simulink library "LiBatteryBlocks"  (Simulink 7.6)
settings: Solver=ode45  StartTime=0.0  StopTime=10.0  RelTol=1e-3
values from neighbouring files (symbols this model uses):
  BatteryParams = struct()    [ssc_lithium_battery_80Cells_ini.m]
  numCells = 80    [ssc_lithium_battery_80Cells_ini.m]
libraries: fl_lib x19, LiBatteryBlocks x8, LiBatteryElements_lib x4, nesl_utility x3
settings Model: Creator=jgazzarr  LastModifiedBy=rjackey

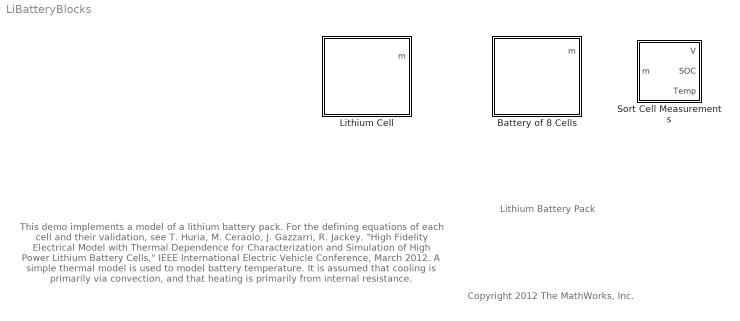
== system LiBatteryBlocks ==
  note: Lithium Battery Pack
  note: This demo implements a model of a lithium battery pack. For the defining equations of each cell and their validation, see T. Huria, M. Ceraolo,
      | J. Gazzarri, R. Jackey. "High Fidelity Electrical Model with Thermal Dependence for Characterization and Simulation of High Power Lithium
      | Battery Cells," IEEE International Electric Vehicle Conference, March 2012. A simple thermal model is used to model battery temperature. It is
      | assumed that cooling is primarily via convection, and that heating is primarily from internal resistance.
  note: Copyright 2012 The MathWorks, Inc.
  Battery of 8 Cells : Subsystem  mask(Battery 8 Series Cells){ThisStackParams=BatteryParams(1:8)}
      mask prompts: ThisStackParams "Parameter Structure (this stack of cells)"
      settings: AttributesFormatString=%<ThisStackParams>
  Lithium Cell : Subsystem  mask(Battery Cell){Battery=BatteryParams(1)}
      mask prompts: Battery "Battery Parameter Structure"
      settings: AttributesFormatString=%<Battery>
      mask Display:
      | image(imread('battery.jpg'))
      | color('red')
      | port_label('LConn',2,'-')
      | port_label('LConn',1,'+')
      | port_label('RConn',1,'H')
      | port_label('output',1,'m')
  Sort Cell Measurements : Subsystem

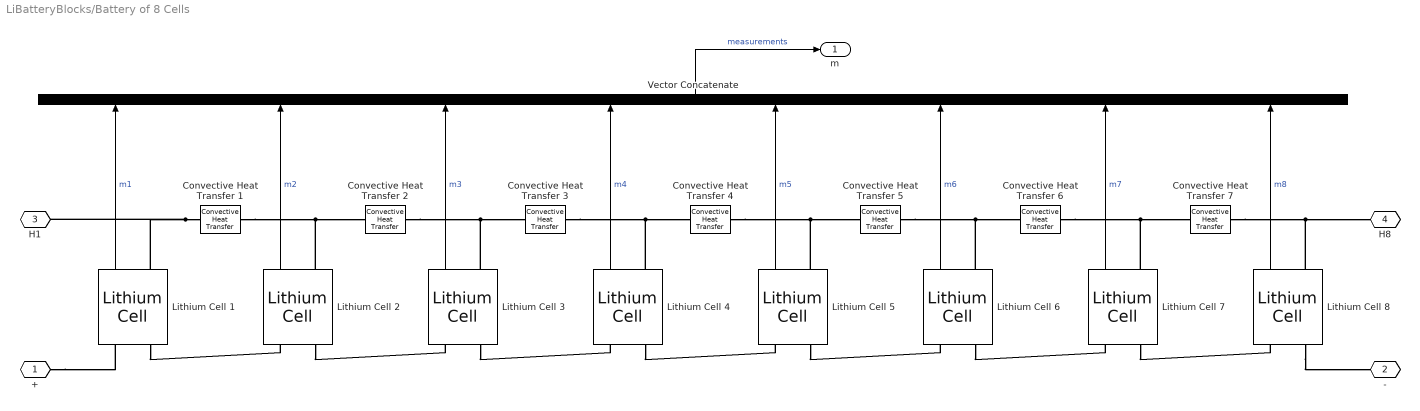
== system LiBatteryBlocks/Battery of 8 Cells ==
  Convective Heat Transfer {1..7} (7 alike) : fl_lib/Thermal/Thermal Elements/Convective Heat Transfer  DialogController=NetworkEngine.DynNeDlgSource  SystemSampleTime=-1  area=cell_area m^2  heat_tr_coeff=h_conv W/(m^2 * K)  Q_Log=off  T_Log=off  LocalVarNames=|heat_flow|temperature_diff  LocalVarDescs=|Heat flow (J/s)|Temperature difference (K)  LocalVarLogging=[0 0]
  Lithium Cell 1 : LiBatteryBlocks/Lithium Cell  SystemSampleTime=-1  Battery=ThisStackParams(1)
      settings: AttributesFormatString=%<Battery>
  Lithium Cell 2 : LiBatteryBlocks/Lithium Cell  SystemSampleTime=-1  Battery=ThisStackParams(2)
      settings: AttributesFormatString=%<Battery>
  Lithium Cell 3 : LiBatteryBlocks/Lithium Cell  SystemSampleTime=-1  Battery=BatteryParams(3)
      settings: AttributesFormatString=%<Battery>
  Lithium Cell 4 : LiBatteryBlocks/Lithium Cell  SystemSampleTime=-1  Battery=ThisStackParams(4)
      settings: AttributesFormatString=%<Battery>
  Lithium Cell 5 : LiBatteryBlocks/Lithium Cell  SystemSampleTime=-1  Battery=ThisStackParams(5)
      settings: AttributesFormatString=%<Battery>
  Lithium Cell 6 : LiBatteryBlocks/Lithium Cell  SystemSampleTime=-1  Battery=ThisStackParams(6)
      settings: AttributesFormatString=%<Battery>
  Lithium Cell 7 : LiBatteryBlocks/Lithium Cell  SystemSampleTime=-1  Battery=ThisStackParams(7)
      settings: AttributesFormatString=%<Battery>
  Lithium Cell 8 : LiBatteryBlocks/Lithium Cell  SystemSampleTime=-1  Battery=ThisStackParams(8)
      settings: AttributesFormatString=%<Battery>
  Vector Concatenate : Concatenate  NumInputs=8  Mode=Vector
  + : PMIOPort  Port=1  Side=Left
  - : PMIOPort  Port=2  Side=Left
  H1 : PMIOPort  Port=3  Side=Right
  H8 : PMIOPort  Port=4  Side=Right
  m : Outport
  wires:
  Lithium Cell 1/1 -> Vector Concatenate/1  "m1"
  Lithium Cell 2/1 -> Vector Concatenate/2  "m2"
  Lithium Cell 3/1 -> Vector Concatenate/3  "m3"
  Lithium Cell 4/1 -> Vector Concatenate/4  "m4"
  Lithium Cell 5/1 -> Vector Concatenate/5  "m5"
  Lithium Cell 6/1 -> Vector Concatenate/6  "m6"
  Lithium Cell 7/1 -> Vector Concatenate/7  "m7"
  Lithium Cell 8/1 -> Vector Concatenate/8  "m8"
  Vector Concatenate/1 -> m/1  "measurements"
  connections:
  Lithium Cell 8/RConn1 -- H8/RConn1 -- Convective Heat Transfer 7/RConn1
  Convective Heat Transfer 1/LConn1 -- H1/RConn1 -- Lithium Cell 1/RConn1
  Lithium Cell 7/LConn2 -- Lithium Cell 8/LConn1
  Lithium Cell 6/LConn2 -- Lithium Cell 7/LConn1
  Lithium Cell 5/LConn2 -- Lithium Cell 6/LConn1
  Lithium Cell 4/LConn2 -- Lithium Cell 5/LConn1
  Lithium Cell 3/LConn2 -- Lithium Cell 4/LConn1
  Lithium Cell 2/LConn2 -- Lithium Cell 3/LConn1
  Lithium Cell 1/LConn2 -- Lithium Cell 2/LConn1
  Lithium Cell 8/LConn2 -- -/RConn1
  Lithium Cell 2/RConn1 -- Convective Heat Transfer 2/LConn1 -- Convective Heat Transfer 1/RConn1
  Lithium Cell 3/RConn1 -- Convective Heat Transfer 3/LConn1 -- Convective Heat Transfer 2/RConn1
  Lithium Cell 4/RConn1 -- Convective Heat Transfer 4/LConn1 -- Convective Heat Transfer 3/RConn1
  Lithium Cell 5/RConn1 -- Convective Heat Transfer 5/LConn1 -- Convective Heat Transfer 4/RConn1
  Lithium Cell 6/RConn1 -- Convective Heat Transfer 6/LConn1 -- Convective Heat Transfer 5/RConn1
  Lithium Cell 7/RConn1 -- Convective Heat Transfer 7/LConn1 -- Convective Heat Transfer 6/RConn1
  +/RConn1 -- Lithium Cell 1/LConn1

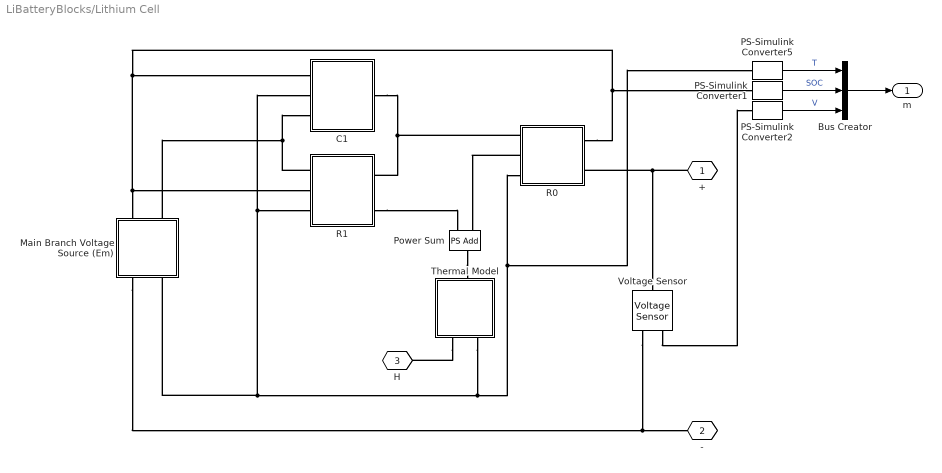
== system LiBatteryBlocks/Lithium Cell ==
  Bus Creator : BusCreator  Inputs=3
  C1 : Subsystem
  Main Branch Voltage Source (Em) : Subsystem
  PS-Simulink Converter1 : nesl_utility/PS-Simulink Converter  DialogController=NetworkEngine.DynNeUtilDlgSource  SystemSampleTime=-1  PhysicalDomain=network_engine_domain  LeftPortType=input  RightPortType=output  SubClassName=ps_output  Unit=1  AffineConversion=off
  PS-Simulink Converter2 : nesl_utility/PS-Simulink Converter  DialogController=NetworkEngine.DynNeUtilDlgSource  SystemSampleTime=-1  PhysicalDomain=network_engine_domain  LeftPortType=input  RightPortType=output  SubClassName=ps_output  Unit=V  AffineConversion=off
  PS-Simulink Converter5 : nesl_utility/PS-Simulink Converter  DialogController=NetworkEngine.DynNeUtilDlgSource  SystemSampleTime=-1  PhysicalDomain=network_engine_domain  LeftPortType=input  RightPortType=output  SubClassName=ps_output  Unit=C  AffineConversion=on
  Power Sum : fl_lib/Physical Signals/Functions/PS Add  DialogController=NetworkEngine.DynNeDlgSource  SystemSampleTime=-1  LocalVarLogging=[]
  R0 : Subsystem
  R1 : Subsystem
  Thermal Model : Subsystem
  Voltage Sensor : fl_lib/Electrical/Electrical Sensors/Voltage Sensor  DialogController=NetworkEngine.DynNeDlgSource  SystemSampleTime=-1  i1_Log=off  v1_Log=off  LocalVarNames=|i1|v1  LocalVarDescs=|i1|v1  LocalVarLogging=[0 0]
  + : PMIOPort  Tag=PMCPort  Port=1  Side=Left
  - : PMIOPort  Tag=PMCPort  Port=2  Side=Left
  H : PMIOPort  Tag=PMCPort  Port=3  Side=Right
  m : Outport
  wires:
  PS-Simulink Converter5/1 -> Bus Creator/1  "T"
  PS-Simulink Converter1/1 -> Bus Creator/2  "SOC"
  Bus Creator/1 -> m/1
  PS-Simulink Converter2/1 -> Bus Creator/3  "V"
  connections:
  R0/RConn1 -- C1/LConn1 -- R1/LConn2 -- Main Branch Voltage Source (Em)/LConn1 -- PS-Simulink Converter1/LConn1
  R1/LConn1 -- Main Branch Voltage Source (Em)/LConn2 -- C1/LConn3
  Thermal Model/RConn2 -- R1/LConn3 -- C1/LConn2 -- Main Branch Voltage Source (Em)/RConn2 -- R0/LConn3 -- PS-Simulink Converter5/LConn1
  R0/LConn1 -- C1/RConn1 -- R1/RConn1
  Power Sum/RConn1 -- Thermal Model/LConn1
  R0/LConn2 -- Power Sum/LConn1
  R1/RConn2 -- Power Sum/LConn2
  +/RConn1 -- R0/RConn2 -- Voltage Sensor/LConn1
  Main Branch Voltage Source (Em)/RConn1 -- -/RConn1 -- Voltage Sensor/RConn2
  Thermal Model/RConn1 -- H/RConn1
  Voltage Sensor/RConn1 -- PS-Simulink Converter2/LConn1

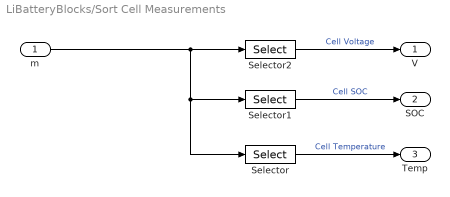
== system LiBatteryBlocks/Sort Cell Measurements ==
  m : Inport
  Selector : Selector  InputPortWidth=numCells * 3  IndexOptions=Index vector (dialog)  Indices=1:3:numCells*3  OutputSizes=1
  Selector1 : Selector  InputPortWidth=numCells * 3  IndexOptions=Index vector (dialog)  Indices=2:3:numCells*3  OutputSizes=1
  Selector2 : Selector  InputPortWidth=numCells * 3  IndexOptions=Index vector (dialog)  Indices=3:3:numCells*3  OutputSizes=1
  V : Outport
  SOC : Outport  Port=2
  Temp : Outport  Port=3
  wires:
  Selector2/1 -> V/1  "Cell Voltage"
  Selector1/1 -> SOC/1  "Cell SOC"
  Selector/1 -> Temp/1  "Cell Temperature"
  m/1 -> Selector1/1, Selector/1, Selector2/1

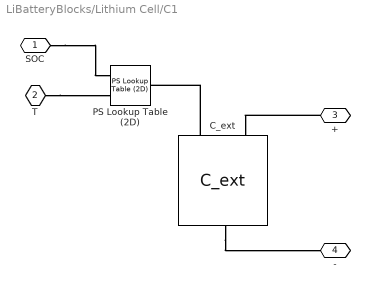
== system LiBatteryBlocks/Lithium Cell/C1 ==
  C_ext : LiBatteryElements_lib/C_ext  DialogController=NetworkEngine.DynNeDlgSource  SystemSampleTime=-1  v0=0 V  Cmin=1e-6 F  i_Log=off  v_Log=off  LocalVarNames=|i|v  LocalVarDescs=|i|v  LocalVarLogging=[0 0]
  PS Lookup Table (2D) : fl_lib/Physical Signals/Lookup Tables/PS Lookup Table (2D)  DialogController=NetworkEngine.DynNeDlgSource  SystemSampleTime=-1  x_t=Battery.SOC_LUT  y_t=Battery.Temperature_LUT  z_t=Battery.C1_LUT  interp_method=1  extrap_method=1  dbg=0  LocalVarLogging=[]
  SOC : PMIOPort  Port=1  Side=Left
  T : PMIOPort  Port=2  Side=Left
  + : PMIOPort  Port=3  Side=Left
  - : PMIOPort  Port=4  Side=Right
  connections:
  +/RConn1 -- C_ext/LConn1
  C_ext/RConn1 -- -/RConn1
  C_ext/LConn2 -- PS Lookup Table (2D)/RConn1
  T/RConn1 -- PS Lookup Table (2D)/LConn2
  SOC/RConn1 -- PS Lookup Table (2D)/LConn1

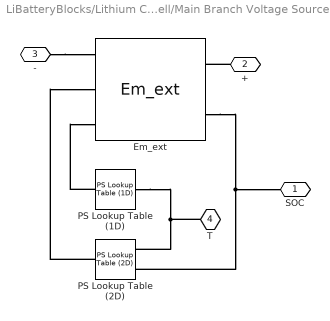
== system LiBatteryBlocks/Lithium Cell/Main Branch Voltage Source (Em) ==
  Em_ext : LiBatteryElements_lib/Em_ext  DialogController=NetworkEngine.DynNeDlgSource  SystemSampleTime=-1  Qinit=Battery.Qe_init hr*A  i_Log=off  v_Log=off  Qe_Log=off  LocalVarNames=|i|v|Qe  LocalVarDescs=|i|v|Extracted charge  LocalVarLogging=[0 0 0]
  PS Lookup Table (1D) : fl_lib/Physical Signals/Lookup Tables/PS Lookup Table (1D)  DialogController=NetworkEngine.DynNeDlgSource  SystemSampleTime=-1  x_t=Battery.Temperature_LUT  y_t=Battery.Capacity_LUT  interp_method=1  extrap_method=1  dbg=0  LocalVarLogging=[]
  PS Lookup Table (2D) : fl_lib/Physical Signals/Lookup Tables/PS Lookup Table (2D)  DialogController=NetworkEngine.DynNeDlgSource  SystemSampleTime=-1  x_t=Battery.SOC_LUT  y_t=Battery.Temperature_LUT  z_t=Battery.Em_LUT  interp_method=1  extrap_method=1  dbg=0  LocalVarLogging=[]
  SOC : PMIOPort  Port=1  Side=Left
  + : PMIOPort  Port=2  Side=Left
  - : PMIOPort  Port=3  Side=Right
  T : PMIOPort  Port=4  Side=Right
  connections:
  PS Lookup Table (1D)/RConn1 -- Em_ext/RConn3
  T/RConn1 -- PS Lookup Table (2D)/LConn2 -- PS Lookup Table (1D)/LConn1
  PS Lookup Table (2D)/RConn1 -- Em_ext/RConn2
  PS Lookup Table (2D)/LConn1 -- SOC/RConn1 -- Em_ext/LConn2
  +/RConn1 -- Em_ext/LConn1
  -/RConn1 -- Em_ext/RConn1

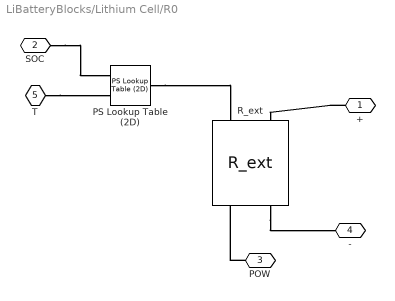
== system LiBatteryBlocks/Lithium Cell/R0 ==
  PS Lookup Table (2D) : fl_lib/Physical Signals/Lookup Tables/PS Lookup Table (2D)  DialogController=NetworkEngine.DynNeDlgSource  SystemSampleTime=-1  x_t=Battery.SOC_LUT  y_t=Battery.Temperature_LUT  z_t=Battery.R0_LUT  interp_method=1  extrap_method=1  dbg=0  LocalVarLogging=[]
  R_ext : LiBatteryElements_lib/R_ext  DialogController=NetworkEngine.DynNeDlgSource  SystemSampleTime=-1  Rmin=0 Ohm  i_Log=off  v_Log=off  LocalVarNames=|i|v  LocalVarDescs=|i|v  LocalVarLogging=[0 0]
  + : PMIOPort  Port=1  Side=Left
  SOC : PMIOPort  Port=2  Side=Right
  POW : PMIOPort  Port=3  Side=Left
  - : PMIOPort  Port=4  Side=Right
  T : PMIOPort  Port=5  Side=Left
  connections:
  SOC/RConn1 -- PS Lookup Table (2D)/LConn1
  PS Lookup Table (2D)/RConn1 -- R_ext/LConn2
  POW/RConn1 -- R_ext/RConn2
  R_ext/RConn1 -- -/RConn1
  +/RConn1 -- R_ext/LConn1
  T/RConn1 -- PS Lookup Table (2D)/LConn2

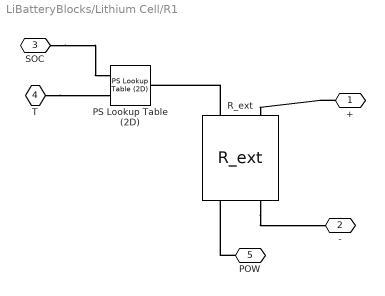
== system LiBatteryBlocks/Lithium Cell/R1 ==
  PS Lookup Table (2D) : fl_lib/Physical Signals/Lookup Tables/PS Lookup Table (2D)  DialogController=NetworkEngine.DynNeDlgSource  SystemSampleTime=-1  x_t=Battery.SOC_LUT  y_t=Battery.Temperature_LUT  z_t=Battery.R1_LUT  interp_method=1  extrap_method=1  dbg=0  LocalVarLogging=[]
  R_ext : LiBatteryElements_lib/R_ext  DialogController=NetworkEngine.DynNeDlgSource  SystemSampleTime=-1  Rmin=0 Ohm  i_Log=off  v_Log=off  LocalVarNames=|i|v  LocalVarDescs=|i|v  LocalVarLogging=[0 0]
  + : PMIOPort  Port=1  Side=Left
  - : PMIOPort  Port=2  Side=Right
  SOC : PMIOPort  Port=3  Side=Left
  T : PMIOPort  Port=4  Side=Left
  POW : PMIOPort  Port=5  Side=Right
  connections:
  +/RConn1 -- R_ext/LConn1
  R_ext/RConn1 -- -/RConn1
  POW/RConn1 -- R_ext/RConn2
  R_ext/LConn2 -- PS Lookup Table (2D)/RConn1
  T/RConn1 -- PS Lookup Table (2D)/LConn2
  SOC/RConn1 -- PS Lookup Table (2D)/LConn1

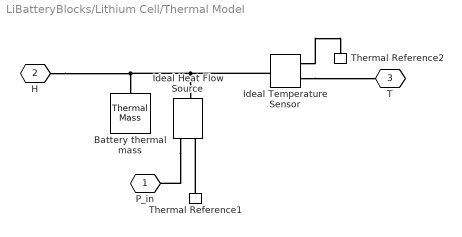
== system LiBatteryBlocks/Lithium Cell/Thermal Model ==
  Battery thermal mass : fl_lib/Thermal/Thermal Elements/Thermal Mass  DialogController=NetworkEngine.DynNeDlgSource  SystemSampleTime=-1  mass=Battery.cell_mass kg  sp_heat=Battery.cell_Cp_heat J/kg/K  init_temp=Battery.T_init K  Q_Log=off  LocalVarNames=|heat_flow|temperature  LocalVarDescs=|Heat flow (J/s)|Mass temperature (K)  LocalVarLogging=[0 0]
  Ideal Temperature Sensor : fl_lib/Thermal/Thermal Sensors/Ideal Temperature Sensor  DialogController=NetworkEngine.DynNeDlgSource  SystemSampleTime=-1  Qs_Log=off  Ts_Log=off  LocalVarNames=|Qs|Ts  LocalVarDescs=|Qs|Ts  LocalVarLogging=[]
  Ideal Heat Flow Source : fl_lib/Thermal/Thermal Sources/Ideal Heat Flow Source  DialogController=NetworkEngine.DynNeDlgSource  SystemSampleTime=-1  Q_Log=off  T_Log=off  LocalVarNames=|heat_flow|T_differential  LocalVarDescs=|Heat flow through the source (J/s)|Temperature differential across the source (K)  LocalVarLogging=[0 0]
  Thermal Reference1 : fl_lib/Thermal/Thermal Elements/Thermal Reference  DialogController=NetworkEngine.DynNeDlgSource  SystemSampleTime=-1  Q_Log=off  LocalVarNames=|Q  LocalVarDescs=|Q  LocalVarLogging=[]
  Thermal Reference2 : fl_lib/Thermal/Thermal Elements/Thermal Reference  DialogController=NetworkEngine.DynNeDlgSource  SystemSampleTime=-1  Q_Log=off  LocalVarNames=|Q  LocalVarDescs=|Q  LocalVarLogging=[]
  P_in : PMIOPort  Tag=PMCPort  Port=1  Side=Left
  H : PMIOPort  Tag=PMCPort  Port=2  Side=Right
  T : PMIOPort  Tag=PMCPort  Port=3  Side=Right
  connections:
  Ideal Heat Flow Source/RConn1 -- P_in/RConn1
  Ideal Heat Flow Source/LConn1 -- Battery thermal mass/LConn1 -- H/RConn1 -- Ideal Temperature Sensor/LConn1
  Thermal Reference1/LConn1 -- Ideal Heat Flow Source/RConn2
  Ideal Temperature Sensor/RConn2 -- T/RConn1
  Ideal Temperature Sensor/RConn1 -- Thermal Reference2/LConn1
